simulink model "TestController2"  (R2023a)
settings: Solver=ode1  StartTime=0.0  StopTime=180  FixedStep=0.001  RelTol=1e-3
values from neighbouring files (symbols this model uses):
  a = 1    [controller_design.m]    (also in controller_test.m = Ks(1).a; find_opt.m = a + 0.1; show_results.m = Ks(1).a)
  b = 1.5    [controller_design.m]    (also in controller_test.m = Ks(1).b; find_opt.m = b + 0.1; show_results.m = Ks(1).b)
  K_I = K_P    [controller_design.m]    (also in controller_test.m = Ks(1).KP_KI; show_results.m = Ks(1).KP_KI)
  K_P = Ks(index).KP_KI    [controller_design.m]    (also in controller_test.m = K_I; show_results.m = K_I)
  Pos_ref_vals = unique(data.Pos_ref)    [InitTestBench.m]
  Q_vals = [0:0.5:13]    [InitTestBench.m]
  R_clamp_mean = mean(R_clamp,2,"omitnan")    [InitTestBench.m]
  v_ref_vals = unique(data.v_ref)    [InitTestBench.m]
settings Model: Creator=borchers  LastModifiedBy=nptlinh

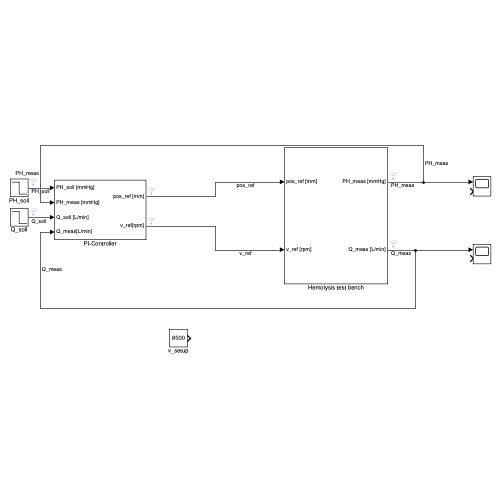
[thumbnail: Simulink's stored preview of the top-level diagram]
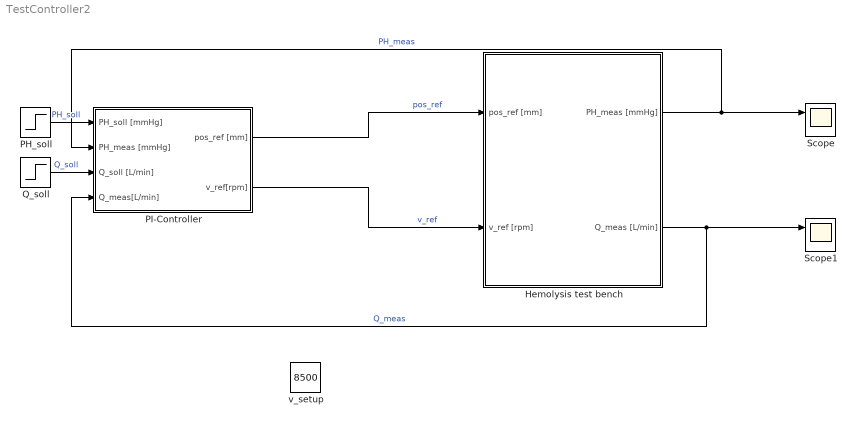
== system TestController2 ==
  Hemolysis test bench : Subsystem
  PH_soll : Step  Time=120  Before=32  After=27.65  SampleTime=0
  PI-Controller : Subsystem
  Q_soll : Step  Time=120  Before=7.25  After=6.75  SampleTime=0
  Scope : Scope  NumInputPorts=2
  Scope1 : Scope  NumInputPorts=2
  v_setup : Constant  Value=8500
  wires:
  Hemolysis test bench/2(Q_meas [L/min]) -> Scope1/1, PI-Controller/4(Q_meas[L/min])  "Q_meas"
  Hemolysis test bench/1(PH_meas [mmHg]) -> PI-Controller/2(PH_meas [mmHg]), Scope/1  "PH_meas"
  PI-Controller/1(pos_ref [mm]) -> Hemolysis test bench/1(pos_ref [mm])  "pos_ref"
  PI-Controller/2(v_ref[rpm]) -> Hemolysis test bench/2(v_ref [rpm])  "v_ref"
  PH_soll/1 -> PI-Controller/1(PH_soll [mmHg])  "PH_soll"
  Q_soll/1 -> PI-Controller/3(Q_soll [L/min])  "Q_soll"

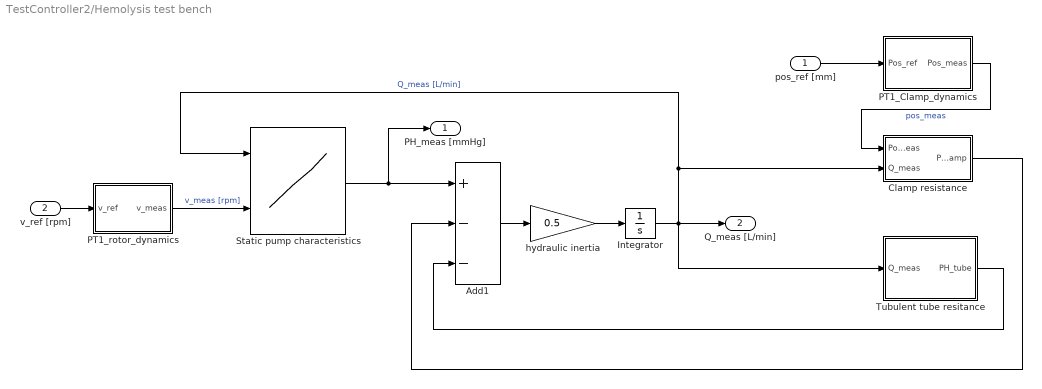
== system TestController2/Hemolysis test bench ==
  pos_ref [mm] : Inport
  v_ref [rpm] : Inport  Port=2
  Add1 : Sum  Inputs=+--
  Clamp resistance : Subsystem
  Integrator : Integrator  InitialCondition=0.01  LimitOutput=on  LowerSaturationLimit=0.01
  PT1_Clamp_dynamics : Subsystem
  PT1_rotor_dynamics : Subsystem
  Static pump characteristics : Lookup_n-D  BreakpointsForDimension1=Q_vals  BreakpointsForDimension2=v_ref_vals  Table=LUT_Static_Pump'  InternalRulePriority=Speed  RndMeth=Simplest
      settings: InputPortMap=u0,u1
  Tubulent tube resitance : Subsystem
  hydraulic inertia : Gain  Gain=0.5
  PH_meas [mmHg] : Outport
  Q_meas [L/min] : Outport  Port=2
  wires:
  Integrator/1 -> Static pump characteristics/1, Clamp resistance/2(Q_meas), Q_meas [L/min]/1, Tubulent tube resitance/1(Q_meas)  "Q_meas [L/min]"
  PT1_rotor_dynamics/1(v_meas) -> Static pump characteristics/2  "v_meas [rpm]"
  v_ref [rpm]/1 -> PT1_rotor_dynamics/1(v_ref)
  pos_ref [mm]/1 -> PT1_Clamp_dynamics/1(Pos_ref)
  Static pump characteristics/1 -> PH_meas [mmHg]/1, Add1/1
  Add1/1 -> hydraulic inertia/1
  hydraulic inertia/1 -> Integrator/1
  Tubulent tube resitance/1(PH_tube) -> Add1/3
  PT1_Clamp_dynamics/1(Pos_meas) -> Clamp resistance/1(Pos_meas)  "pos_meas"
  Clamp resistance/1(PH_clamp) -> Add1/2

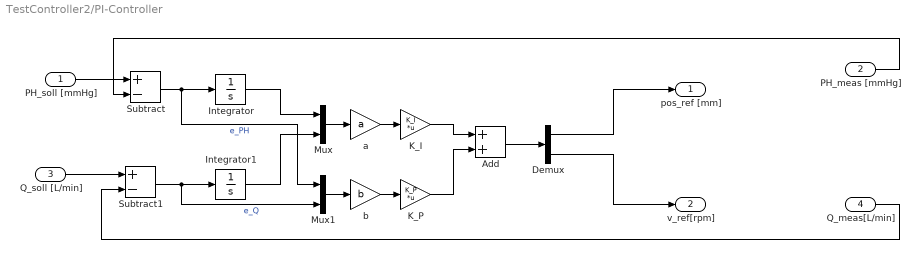
== system TestController2/PI-Controller ==
  PH_soll [mmHg] : Inport
  PH_meas [mmHg] : Inport  Port=2
  Q_soll [L/min] : Inport  Port=3
  Q_meas[L/min] : Inport  Port=4
  Add : Sum
  Demux : Demux  Outputs=2
  Integrator : Integrator
  Integrator1 : Integrator
  K_I : Gain  Gain=K_I  Multiplication=Matrix(K*u)
  K_P : Gain  Gain=K_P  Multiplication=Matrix(K*u)
  Mux : Mux  Inputs=2
  Mux1 : Mux  Inputs=2
  Subtract : Sum  Inputs=+-
  Subtract1 : Sum  Inputs=+-
  a : Gain  Gain=a
  b : Gain  Gain=b
  pos_ref [mm] : Outport
  v_ref[rpm] : Outport  Port=2
  wires:
  Q_meas[L/min]/1 -> Subtract1/2
  PH_soll [mmHg]/1 -> Subtract/1
  Integrator1/1 -> Mux/2
  Integrator/1 -> Mux/1
  PH_meas [mmHg]/1 -> Subtract/2
  Demux/2 -> v_ref[rpm]/1
  Subtract/1 -> Mux1/1, Integrator/1  "e_PH"
  Q_soll [L/min]/1 -> Subtract1/1
  Demux/1 -> pos_ref [mm]/1
  Subtract1/1 -> Mux1/2, Integrator1/1  "e_Q"
  Add/1 -> Demux/1
  K_I/1 -> Add/1
  K_P/1 -> Add/2
  Mux/1 -> a/1
  a/1 -> K_I/1
  Mux1/1 -> b/1
  b/1 -> K_P/1

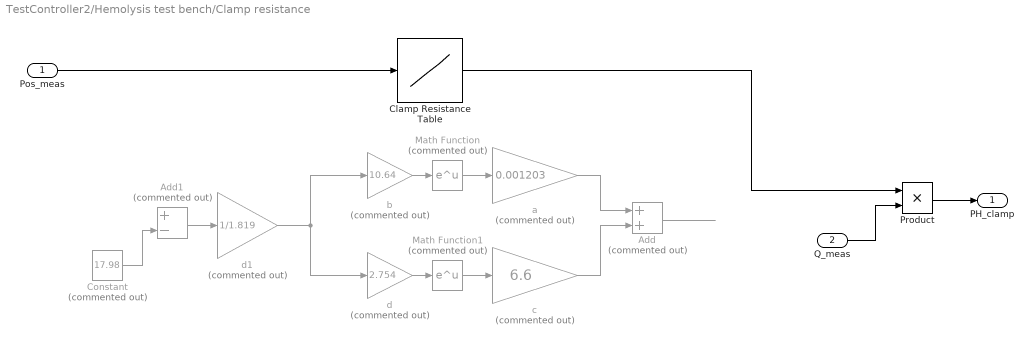
== system TestController2/Hemolysis test bench/Clamp resistance ==
  Pos_meas : Inport
  Q_meas : Inport  Port=2
  Add : Sum  Commented=on
  Add1 : Sum  Commented=on  Inputs=+-
  Clamp Resistance Table : Lookup_n-D  NumberOfTableDimensions=1  BreakpointsForDimension1=Pos_ref_vals  Table=R_clamp_mean  InternalRulePriority=Speed  RndMeth=Simplest
  Constant : Constant  Commented=on  Value=17.98
  Math Function : Math  Commented=on
  Math Function1 : Math  Commented=on
  Product : Product
  a : Gain  Commented=on  Gain=0.001203
  b : Gain  Commented=on  Gain=10.64
  c : Gain  Commented=on  Gain=6.6
  d : Gain  Commented=on  Gain=2.754
  d1 : Gain  Commented=on  Gain=1/1.819
  PH_clamp : Outport
  wires:
  Product/1 -> PH_clamp/1
  Q_meas/1 -> Product/2
  Math Function/1 -> a/1
  b/1 -> Math Function/1
  a/1 -> Add/1
  d1/1 -> d/1, b/1
  c/1 -> Add/2
  d/1 -> Math Function1/1
  Math Function1/1 -> c/1
  Add1/1 -> d1/1
  Constant/1 -> Add1/2
  Pos_meas/1 -> Clamp Resistance Table/1
  Add/1 -> ?
  Clamp Resistance Table/1 -> Product/1

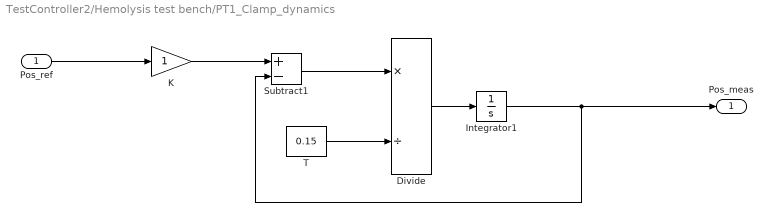
== system TestController2/Hemolysis test bench/PT1_Clamp_dynamics ==
  Pos_ref : Inport
  Divide : Product  Inputs=*/
  Integrator1 : Integrator  InitialCondition=18
  K : Gain
  Subtract1 : Sum  Inputs=+-
  T : Constant  Value=0.15
  Pos_meas : Outport
  wires:
  Divide/1 -> Integrator1/1
  Pos_ref/1 -> K/1
  K/1 -> Subtract1/1
  Subtract1/1 -> Divide/1
  T/1 -> Divide/2
  Integrator1/1 -> Pos_meas/1, Subtract1/2

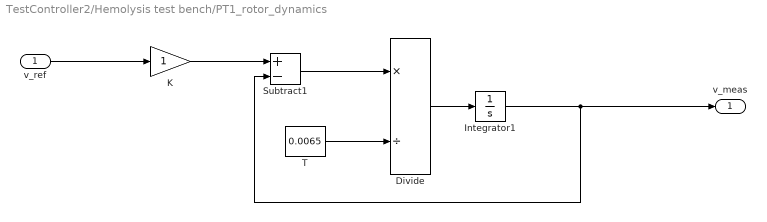
== system TestController2/Hemolysis test bench/PT1_rotor_dynamics ==
  v_ref : Inport
  Divide : Product  Inputs=*/
  Integrator1 : Integrator  InitialCondition=11000
  K : Gain
  Subtract1 : Sum  Inputs=+-
  T : Constant  Value=0.0065
  v_meas : Outport
  wires:
  Divide/1 -> Integrator1/1
  v_ref/1 -> K/1
  Integrator1/1 -> v_meas/1, Subtract1/2
  K/1 -> Subtract1/1
  Subtract1/1 -> Divide/1
  T/1 -> Divide/2

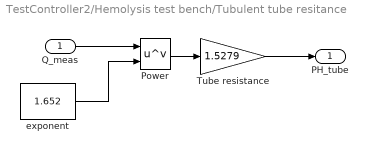
== system TestController2/Hemolysis test bench/Tubulent tube resitance ==
  Q_meas : Inport
  Power : Math  Operator=pow
  Tube resistance : Gain  Gain=1.5279
  exponent : Constant  Value=1.652
  PH_tube : Outport
  wires:
  exponent/1 -> Power/2
  Power/1 -> Tube resistance/1
  Q_meas/1 -> Power/1
  Tube resistance/1 -> PH_tube/1
